simulink model "question2"  (R2023b)
settings: Solver=VariableStepAuto  StartTime=0.0  StopTime=10  RelTol=1e-3
values from neighbouring files (symbols this model uses):
  A = [-8.8487+(a-b)/5,-0.0399,-5.55+(c+d)/10,3.5846 ... (first row only)    [main_func.m]    (also in question3.m = [-8.8487+(a-b)/5, -0.0399, -5.55+(c+d)/10, 3.5846)
  B = [0.0564+b/(10+c),0.0319 ... (first row only)    [main_func.m]    (also in question3.m = [0.0564+b/(10+c), 0.0319)
  C = [-3.2988,-2.1932+(10*c+d)/(100+5*a),0.037,-0.0109 ... (first row only)    [main_func.m]    (also in question3.m = [-3.2988, -2.1932+(10*c+d)/(100+5*a), 0.037, -0.0109)
  K2 = lqr(A,B,Q,R)    [main_func.m]    (also in servo_control.m = K(:,5:6); servo_control_state.m = K(:,5:6))
  x0 = [0.5;-0.1;0.3;-0.8]    [main_func.m]    (also in question3.m = [0.5; -0.1; 0.3; -0.8])
settings Model: Creator=Fan Xiuqi  LastModifiedBy=Fan Xiuqi

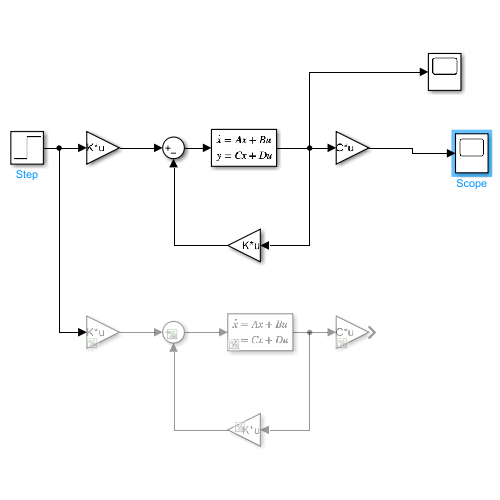
[thumbnail: Simulink's stored preview of the top-level diagram]
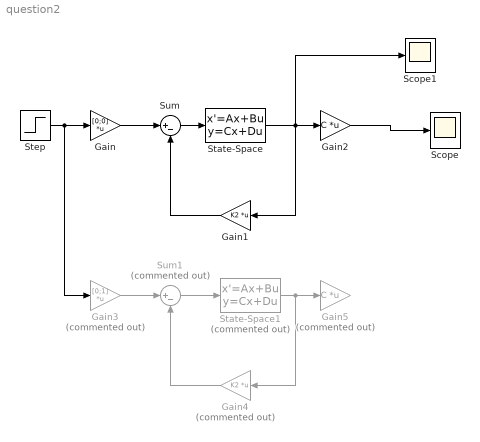
== system question2 ==
  Gain : Gain  Gain=[0;0]  Multiplication=Matrix(K*u)
  Gain1 : Gain  Gain=K2  Multiplication=Matrix(K*u)
  Gain2 : Gain  Gain=C  Multiplication=Matrix(K*u)
  Gain3 : Gain  Commented=on  Gain=[0;1]  Multiplication=Matrix(K*u)
  Gain4 : Gain  Commented=on  Gain=K2  Multiplication=Matrix(K*u)
  Gain5 : Gain  Commented=on  Gain=C  Multiplication=Matrix(K*u)
  Scope : Scope
  Scope1 : Scope
  State-Space : StateSpace  A=A  B=B  C=eye(4)  D=zeros(4,2)  InitialCondition=x0
  State-Space1 : StateSpace  Commented=on  A=A  B=B  C=eye(4)  D=zeros(4,2)  InitialCondition=0
  Step : Step  SampleTime=0
  Sum : Sum  Inputs=|+-
  Sum1 : Sum  Commented=on  Inputs=|+-
  wires:
  Step/1 -> Gain3/1, Gain/1
  Gain/1 -> Sum/1
  Sum/1 -> State-Space/1
  Gain2/1 -> Scope/1
  State-Space/1 -> Scope1/1, Gain2/1, Gain1/1
  Gain1/1 -> Sum/2
  State-Space1/1 -> Gain5/1, Gain4/1
  Sum1/1 -> State-Space1/1
  Gain3/1 -> Sum1/1
  Gain4/1 -> Sum1/2
